simulink library "mpc555phytec"  (Simulink 6.0)
settings: Solver=ode45  SolverMode=SingleTasking  StartTime=0.0  StopTime=10.0  RelTol=1e-3
libraries: target_mpc555 x2
settings Model: Creator=The MathWorks Inc.  LastModifiedBy=batserve  ExtModeAutoUpdateStatusClock=off
settings OptimizationCC: BooleanDataType=off
settings DebuggingCC: CheckExecutionContextPreStartOutputMsg=on  CheckExecutionContextRuntimeOutputMsg=on  SolverPrmCheckMsg=none
settings HardwareCC: TargetUnknown=on

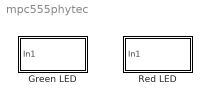
== system mpc555phytec ==
  Green LED : Subsystem  PropExecContextAcrossSSBoundary=on
      mask Type: Green LED
      mask Description: Green LED
      mask Help: Green LED
      mask Display: disp('Green LED')
  Red LED : Subsystem  PropExecContextAcrossSSBoundary=on
      mask Type: Red LED
      mask Description: Red LED
      mask Help: Red LED
      mask Display: disp('Red LED')

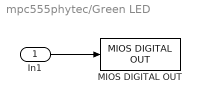
== system mpc555phytec/Green LED ==
  In1 : Inport  Port=1  LatchInput=off
  MIOS DIGITAL OUT : target_mpc555/MIOS/MIOS DIGITAL OUT  bits=0  enablePassThru=off
  wires:
  In1/1 -> MIOS DIGITAL OUT/1

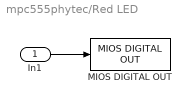
== system mpc555phytec/Red LED ==
  In1 : Inport  Port=1  LatchInput=off
  MIOS DIGITAL OUT : target_mpc555/MIOS/MIOS DIGITAL OUT  bits=1  enablePassThru=off
  wires:
  In1/1 -> MIOS DIGITAL OUT/1
